simulink library "mbd_s32k_examples"  (Simulink 9.0)
settings: Solver=FixedStepDiscrete  StartTime=0.0  StopTime=10.0  FixedStep=0.1  RelTol=1e-3  EnableMultiTasking=on
InitFcn:
  | mbd_s32k14_consistency_checks(bdroot(gcs));
(part 2 of 3)

== system mbd_s32k_examples/S32K11x MCU Simulink Models/Communications Modules/CAN ==
  CAN_Echo : Subsystem  mask{A=[]}
      mask prompts: A "Needed to invoke OpenFcn from the browser:"
      settings: OpenFcn=sfundemo_open('flexcan_echo_s32k11x')
      mask Display: disp('FlexCAN\nEcho');
  CAN_FD_Master : Subsystem  mask{A=[]}
      mask prompts: A "Needed to invoke OpenFcn from the browser:"
      settings: OpenFcn=sfundemo_open('flexcan_can_fd_master_s32k11x')
      mask Display: disp('FlexCAN\nFD Master');
  CAN_FD_Slave : Subsystem  mask{A=[]}
      mask prompts: A "Needed to invoke OpenFcn from the browser:"
      settings: OpenFcn=sfundemo_open('flexcan_can_fd_slave_s32k11x')
      mask Display: disp('FlexCAN\nFD Slave');
  CAN_Loopback : Subsystem  mask{A=[]}
      mask prompts: A "Needed to invoke OpenFcn from the browser:"
      settings: OpenFcn=sfundemo_open('flexcan_loopback_s32k11x')
      mask Display: disp('FlexCAN\nLoopback');
  CAN_Master_XFER : Subsystem  mask{A=[]}
      mask prompts: A "Needed to invoke OpenFcn from the browser:"
      settings: OpenFcn=sfundemo_open('flexcan_master_xfer_status_s32k11x')
      mask Display: disp('FlexCAN\nMaster XFER');
  CAN_Traffic : Subsystem  mask{A=[]}
      mask prompts: A "Needed to invoke OpenFcn from the browser:"
      settings: OpenFcn=sfundemo_open('flexcan_s32k11x')
      mask Display: disp('FlexCAN\nTraffic');

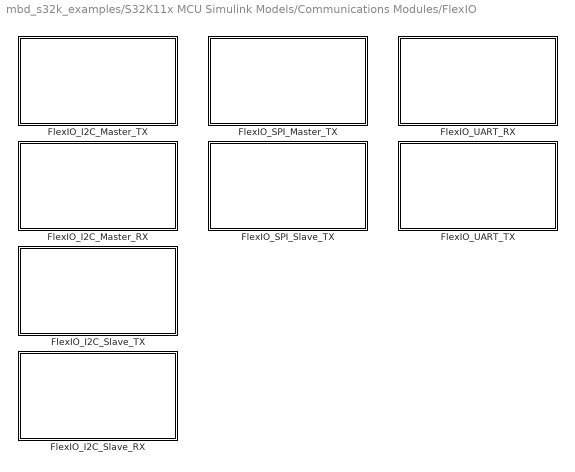
== system mbd_s32k_examples/S32K11x MCU Simulink Models/Communications Modules/FlexIO ==
  FlexIO_I2C_Master_RX : Subsystem  mask{A=[]}
      mask prompts: A "Needed to invoke OpenFcn from the browser:"
      settings: OpenFcn=sfundemo_open('fxio_i2c_master_rx_s32k11x')
      mask Display: disp('FlexIO I2C\nMaster Receive');
  FlexIO_I2C_Master_TX : Subsystem  mask{A=[]}
      mask prompts: A "Needed to invoke OpenFcn from the browser:"
      settings: OpenFcn=sfundemo_open('fxio_i2c_master_tx_s32k11x')
      mask Display: disp('FlexIO I2C\nMaster Transfer');
  FlexIO_I2C_Slave_RX : Subsystem  mask{A=[]}
      mask prompts: A "Needed to invoke OpenFcn from the browser:"
      settings: OpenFcn=sfundemo_open('fxio_i2c_slave_rx_s32k11x')
      mask Display: disp('FlexIO I2C\nSlave Receive');
  FlexIO_I2C_Slave_TX : Subsystem  mask{A=[]}
      mask prompts: A "Needed to invoke OpenFcn from the browser:"
      settings: OpenFcn=sfundemo_open('fxio_i2c_slave_tx_s32k11x')
      mask Display: disp('FlexIO I2C\nSlave Transfer');
  FlexIO_SPI_Master_TX : Subsystem  mask{A=[]}
      mask prompts: A "Needed to invoke OpenFcn from the browser:"
      settings: OpenFcn=sfundemo_open('fxio_spi_master_s32k11x')
      mask Display: disp('FlexIO SPI\nMaster Transfer');
  FlexIO_SPI_Slave_TX : Subsystem  mask{A=[]}
      mask prompts: A "Needed to invoke OpenFcn from the browser:"
      settings: OpenFcn=sfundemo_open('fxio_spi_slave_s32k11x')
      mask Display: disp('FlexIO SPI\nSlave Transfer');
  FlexIO_UART_RX : Subsystem  mask{A=[]}
      mask prompts: A "Needed to invoke OpenFcn from the browser:"
      settings: OpenFcn=sfundemo_open('fxio_uart_receive_isr_s32k11x')
      mask Display: disp('FlexIO UART\nRX');
  FlexIO_UART_TX : Subsystem  mask{A=[]}
      mask prompts: A "Needed to invoke OpenFcn from the browser:"
      settings: OpenFcn=sfundemo_open('fxio_uart_transmit_isr_s32k11x')
      mask Display: disp('FlexIO UART\nTX');

== system mbd_s32k_examples/S32K11x MCU Simulink Models/Communications Modules/I2C ==
  I2C_Master_Request : Subsystem  mask{A=[]}
      mask prompts: A "Needed to invoke OpenFcn from the browser:"
      settings: OpenFcn=sfundemo_open('lpi2c_master_request_s32k11x')
      mask Display: disp('I2C\nMaster Request');
  I2C_Master_Send : Subsystem  mask{A=[]}
      mask prompts: A "Needed to invoke OpenFcn from the browser:"
      settings: OpenFcn=sfundemo_open('lpi2c_master_send_s32k11x')
      mask Display: disp('I2C\nMaster Send');
  I2C_Slave_Receive : Subsystem  mask{A=[]}
      mask prompts: A "Needed to invoke OpenFcn from the browser:"
      settings: OpenFcn=sfundemo_open('lpi2c_slave_recv_s32k11x')
      mask Display: disp('I2C\nSlave Receive');
  I2C_Slave_Send : Subsystem  mask{A=[]}
      mask prompts: A "Needed to invoke OpenFcn from the browser:"
      settings: OpenFcn=sfundemo_open('lpi2c_master_send_s32k11x')
      mask Display: disp('I2C\nSlave Send');

== system mbd_s32k_examples/S32K11x MCU Simulink Models/Communications Modules/SPI ==
  SPI_Master_Slave_Communication : Subsystem  mask{A=[]}
      mask prompts: A "Needed to invoke OpenFcn from the browser:"
      settings: OpenFcn=sfundemo_open('lpspi_master_slave_s32k11x')
      mask Display: disp('SPI\nMaster&Slave\nPing Pong');

== system mbd_s32k_examples/S32K11x MCU Simulink Models/Communications Modules/Serial ==
  UART_Echo : Subsystem  mask{A=[]}
      mask prompts: A "Needed to invoke OpenFcn from the browser:"
      settings: OpenFcn=sfundemo_open('lpuart_s32k11x')
      mask Display: disp('LPUART\nEcho');
  UART_Hello_World : Subsystem  mask{A=[]}
      mask prompts: A "Needed to invoke OpenFcn from the browser:"
      settings: OpenFcn=sfundemo_open('lpuart_hello_world_s32k11x')
      mask Display: disp('UART\nHello World');

== system mbd_s32k_examples/S32K11x MCU Simulink Models/Core & Systems/DMA_Scatter_Gather ==
  Gain : Gain  SaturateOnIntegerOverflow=on  OutDataTypeStr=Inherit: Same as input  ParamDataTypeStr=Inherit: Same as input

== system mbd_s32k_examples/S32K11x MCU Simulink Models/Core & Systems/DMA_Transfer ==
  Gain : Gain  SaturateOnIntegerOverflow=on  OutDataTypeStr=Inherit: Same as input  ParamDataTypeStr=Inherit: Same as input

== system mbd_s32k_examples/S32K11x MCU Simulink Models/Core & Systems/Low_Power_Complex_Counter ==
  Gain : Gain  SaturateOnIntegerOverflow=on  OutDataTypeStr=Inherit: Same as input  ParamDataTypeStr=Inherit: Same as input

== system mbd_s32k_examples/S32K11x MCU Simulink Models/Core & Systems/Low_Power_Pulse_Counter ==
  Gain : Gain  SaturateOnIntegerOverflow=on  OutDataTypeStr=Inherit: Same as input  ParamDataTypeStr=Inherit: Same as input

== system mbd_s32k_examples/S32K11x MCU Simulink Models/Core & Systems/Low_Power_Timer ==
  Gain : Gain  SaturateOnIntegerOverflow=on  OutDataTypeStr=Inherit: Same as input  ParamDataTypeStr=Inherit: Same as input

== system mbd_s32k_examples/S32K11x MCU Simulink Models/Core & Systems/Power_Management_IO ==
  Gain : Gain  SaturateOnIntegerOverflow=on  OutDataTypeStr=Inherit: Same as input  ParamDataTypeStr=Inherit: Same as input

== system mbd_s32k_examples/S32K11x MCU Simulink Models/Core & Systems/Power_Management_ISR ==
  Gain : Gain  SaturateOnIntegerOverflow=on  OutDataTypeStr=Inherit: Same as input  ParamDataTypeStr=Inherit: Same as input

== system mbd_s32k_examples/S32K11x MCU Simulink Models/Core & Systems/Power_Management_Modes ==
  Gain : Gain  SaturateOnIntegerOverflow=on  OutDataTypeStr=Inherit: Same as input  ParamDataTypeStr=Inherit: Same as input

== system mbd_s32k_examples/S32K11x MCU Simulink Models/Core & Systems/RTC_Alarm ==
  Gain : Gain  SaturateOnIntegerOverflow=on  OutDataTypeStr=Inherit: Same as input  ParamDataTypeStr=Inherit: Same as input

== system mbd_s32k_examples/S32K11x MCU Simulink Models/Core & Systems/Watchdog_Reset ==
  Gain : Gain  SaturateOnIntegerOverflow=on  OutDataTypeStr=Inherit: Same as input  ParamDataTypeStr=Inherit: Same as input

== system mbd_s32k_examples/S32K11x MCU Simulink Models/Download in FLASH/FLASH_BAM_S32K116 ==
  Gain : Gain  SaturateOnIntegerOverflow=on  OutDataTypeStr=Inherit: Same as input  ParamDataTypeStr=Inherit: Same as input

== system mbd_s32k_examples/S32K11x MCU Simulink Models/Download in FLASH/FLASH_BAM_S32K118 ==
  Gain : Gain  SaturateOnIntegerOverflow=on  OutDataTypeStr=Inherit: Same as input  ParamDataTypeStr=Inherit: Same as input

== system mbd_s32k_examples/S32K11x MCU Simulink Models/General Purpose IO/GPIO_ISR ==
  Gain : Gain  SaturateOnIntegerOverflow=on  OutDataTypeStr=Inherit: Same as input  ParamDataTypeStr=Inherit: Same as input

== system mbd_s32k_examples/S32K11x MCU Simulink Models/General Purpose IO/GPIO_S32K11xEVB ==
  Gain : Gain  SaturateOnIntegerOverflow=on  OutDataTypeStr=Inherit: Same as input  ParamDataTypeStr=Inherit: Same as input

== system mbd_s32k_examples/S32K11x MCU Simulink Models/Hardware Timers/CAP_Dual_Edge ==
  Gain : Gain  SaturateOnIntegerOverflow=on  OutDataTypeStr=Inherit: Same as input  ParamDataTypeStr=Inherit: Same as input

== system mbd_s32k_examples/S32K11x MCU Simulink Models/Hardware Timers/CAP_Edge ==
  Gain : Gain  SaturateOnIntegerOverflow=on  OutDataTypeStr=Inherit: Same as input  ParamDataTypeStr=Inherit: Same as input

== system mbd_s32k_examples/S32K11x MCU Simulink Models/Hardware Timers/CAP_Quadrature_Counter_Direction ==
  Gain : Gain  SaturateOnIntegerOverflow=on  OutDataTypeStr=Inherit: Same as input  ParamDataTypeStr=Inherit: Same as input

== system mbd_s32k_examples/S32K11x MCU Simulink Models/Hardware Timers/CAP_Quadrature_Phase_Mode ==
  Gain : Gain  SaturateOnIntegerOverflow=on  OutDataTypeStr=Inherit: Same as input  ParamDataTypeStr=Inherit: Same as input

== system mbd_s32k_examples/S32K11x MCU Simulink Models/Hardware Timers/LPIT_Enable_Disable ==
  Gain : Gain  SaturateOnIntegerOverflow=on  OutDataTypeStr=Inherit: Same as input  ParamDataTypeStr=Inherit: Same as input

== system mbd_s32k_examples/S32K11x MCU Simulink Models/Hardware Timers/LPIT_Start_Stop_Modes ==
  Gain : Gain  SaturateOnIntegerOverflow=on  OutDataTypeStr=Inherit: Same as input  ParamDataTypeStr=Inherit: Same as input

== system mbd_s32k_examples/S32K11x MCU Simulink Models/Hardware Timers/LPIT_Timer_Interrupts ==
  Gain : Gain  SaturateOnIntegerOverflow=on  OutDataTypeStr=Inherit: Same as input  ParamDataTypeStr=Inherit: Same as input

== system mbd_s32k_examples/S32K11x MCU Simulink Models/Hardware Timers/PDB_Counter_Interrupts ==
  Gain : Gain  SaturateOnIntegerOverflow=on  OutDataTypeStr=Inherit: Same as input  ParamDataTypeStr=Inherit: Same as input

== system mbd_s32k_examples/S32K11x MCU Simulink Models/Hardware Timers/PWM_Complementary ==
  Gain : Gain  SaturateOnIntegerOverflow=on  OutDataTypeStr=Inherit: Same as input  ParamDataTypeStr=Inherit: Same as input

== system mbd_s32k_examples/S32K11x MCU Simulink Models/Hardware Timers/PWM_Edge_Aligned ==
  Gain : Gain  SaturateOnIntegerOverflow=on  OutDataTypeStr=Inherit: Same as input  ParamDataTypeStr=Inherit: Same as input

== system mbd_s32k_examples/S32K11x MCU Simulink Models/Hardware Timers/PWM_Three_Phase ==
  Gain : Gain  SaturateOnIntegerOverflow=on  OutDataTypeStr=Inherit: Same as input  ParamDataTypeStr=Inherit: Same as input

== system mbd_s32k_examples/S32K11x MCU Simulink Models/Hardware Timers/TOF_Interrupts ==
  Gain : Gain  SaturateOnIntegerOverflow=on  OutDataTypeStr=Inherit: Same as input  ParamDataTypeStr=Inherit: Same as input

== system mbd_s32k_examples/S32K11x MCU Simulink Models/Local Interconnect Network/LIN Master  ==
  Gain : Gain  SaturateOnIntegerOverflow=on  OutDataTypeStr=Inherit: Same as input  ParamDataTypeStr=Inherit: Same as input

== system mbd_s32k_examples/S32K11x MCU Simulink Models/Local Interconnect Network/LIN Slave ==
  Gain : Gain  SaturateOnIntegerOverflow=on  OutDataTypeStr=Inherit: Same as input  ParamDataTypeStr=Inherit: Same as input

== system mbd_s32k_examples/S32K11x MCU Simulink Models/Peripheral Bridge/Memory_Access_RW ==
  Gain : Gain  SaturateOnIntegerOverflow=on  OutDataTypeStr=Inherit: Same as input  ParamDataTypeStr=Inherit: Same as input

== system mbd_s32k_examples/S32K11x MCU Simulink Models/Peripheral Bridge/Register_Access_RW ==
  Gain : Gain  SaturateOnIntegerOverflow=on  OutDataTypeStr=Inherit: Same as input  ParamDataTypeStr=Inherit: Same as input

== system mbd_s32k_examples/S32K11x MCU Simulink Models/System Basis Chips/SBC_RW_Registers ==
  Gain : Gain  SaturateOnIntegerOverflow=on  OutDataTypeStr=Inherit: Same as input  ParamDataTypeStr=Inherit: Same as input

== system mbd_s32k_examples/S32K11x MCU Simulink Models/System Basis Chips/UJA1169_Control ==
  Gain : Gain  SaturateOnIntegerOverflow=on  OutDataTypeStr=Inherit: Same as input  ParamDataTypeStr=Inherit: Same as input

== system mbd_s32k_examples/S32K14x MCU Simulink Models/AMMCLIB/AMCLIB ==
  AMCLIB_BackEMF_OBSERVER_F16 : Subsystem  mask{A=[]}
      mask prompts: A "Needed to invoke OpenFcn from the browser:"
      settings: OpenFcn=sfundemo_open('ammclib_amclib_observer_F16_s32k14x')
      mask Display: disp('OBSERVERS\nBackEMF observer and\nPosition Tracking observer\nexample for F16 datatypes');
  AMCLIB_BackEMF_OBSERVER_F32 : Subsystem  mask{A=[]}
      mask prompts: A "Needed to invoke OpenFcn from the browser:"
      settings: OpenFcn=sfundemo_open('ammclib_amclib_observer_F32_s32k14x')
      mask Display: disp('OBSERVERS\nBackEMF observer and\nPosition Tracking observer\nexample for F32 datatypes');
  AMCLIB_BackEMF_OBSERVER_FLT : Subsystem  mask{A=[]}
      mask prompts: A "Needed to invoke OpenFcn from the browser:"
      settings: OpenFcn=sfundemo_open('ammclib_amclib_observer_FLT_s32k14x')
      mask Display: disp('OBSERVERS\nBackEMF observer and\nPosition Tracking observer\nexample for FLT datatypes');
  AMCLIB_CURRENT_LOOP : Subsystem  mask{A=[]}
      mask prompts: A "Needed to invoke OpenFcn from the browser:"
      settings: OpenFcn=sfundemo_open('ammclib_amclib_current_loop_s32k14x')
      mask Display: disp('CURRENT LOOP\nCurrent Loop FOC\n for F16/F32/FLT datatypes');
  AMCLIB_FW : Subsystem  mask{A=[]}
      mask prompts: A "Needed to invoke OpenFcn from the browser:"
      settings: OpenFcn=sfundemo_open('ammclib_amclib_field_weakening_s32k14x')
      mask Display: disp('FW\nField-Weakening Algorithm\non PMSM examples\n for F16/F32/FLT datatypes');
  AMCLIB_SPEED_LOOP : Subsystem  mask{A=[]}
      mask prompts: A "Needed to invoke OpenFcn from the browser:"
      settings: OpenFcn=sfundemo_open('ammclib_amclib_speed_loop_s32k14x')
      mask Display: disp('SPEED LOOP\nSpeed Loop FOC\n for F16/F32/FLT datatypes');
  AMCLIB_SPEED_LOOP_with_FW : Subsystem  mask{A=[]}
      mask prompts: A "Needed to invoke OpenFcn from the browser:"
      settings: OpenFcn=sfundemo_open('ammclib_amclib_FW_speed_loop_s32k14x')
      mask Display: disp('FW SPEED LOOP\nSpeed Loop with\nField Weakening examples\nfor F16/F32/FLT datatypes');

== system mbd_s32k_examples/S32K14x MCU Simulink Models/AMMCLIB/GDFLIB ==
  GDFLIB_FIR : Subsystem  mask{A=[]}
      mask prompts: A "Needed to invoke OpenFcn from the browser:"
      settings: OpenFcn=sfundemo_open('ammclib_gdflib_fir_s32k14x')
      mask Display: disp('FIR\nFinite Impulse Response filter for\nF16/F32/FLT datatypes');
  GDFLIB_IIR1 : Subsystem  mask{A=[]}
      mask prompts: A "Needed to invoke OpenFcn from the browser:"
      settings: OpenFcn=sfundemo_open('ammclib_gdflib_iir1_s32k14x')
      mask Display: disp('IIR1\nFirst order\nInfinite Impulse Response filter for\nF16/F32/FLT datatypes');
  GDFLIB_IIR2 : Subsystem  mask{A=[]}
      mask prompts: A "Needed to invoke OpenFcn from the browser:"
      settings: OpenFcn=sfundemo_open('ammclib_gdflib_iir2_s32k14x')
      mask Display: disp('IIR2\nSecond order\nInfinite Impulse Response filter for\nF16/F32/FLT datatypes');
  GDFLIB_MA : Subsystem  mask{A=[]}
      mask prompts: A "Needed to invoke OpenFcn from the browser:"
      settings: OpenFcn=sfundemo_open('ammclib_gdflib_ma_s32k14x')
      mask Display: disp('MA\nMoving Average filter for\nF16/F32/FLT datatypes');

== system mbd_s32k_examples/S32K14x MCU Simulink Models/AMMCLIB/GFLIB ==
  GFLIB_LIMIT : Subsystem  mask{A=[]}
      mask prompts: A "Needed to invoke OpenFcn from the browser:"
      settings: OpenFcn=sfundemo_open('ammclib_gflib_limit_s32k14x')
      mask Display: disp('LIMIT\nScalar and Vector\nlimiting examples for\nF16/F32/FLT datatypes');
  GFLIB_LOG : Subsystem  mask{A=[]}
      mask prompts: A "Needed to invoke OpenFcn from the browser:"
      settings: OpenFcn=sfundemo_open('ammclib_gflib_log_s32k14x')
      mask Display: disp('LOG\nLogarithm examples for\nF16/F32/FLT datatypes');
  GFLIB_LUT : Subsystem  mask{A=[]}
      mask prompts: A "Needed to invoke OpenFcn from the browser:"
      settings: OpenFcn=sfundemo_open('ammclib_gflib_lut_s32k14x')
      mask Display: disp('LUT\nLook-up-Tables examples for\nF16/F32/FLT datatypes');
  GFLIB_MISCELLANEOUS : Subsystem  mask{A=[]}
      mask prompts: A "Needed to invoke OpenFcn from the browser:"
      settings: OpenFcn=sfundemo_open('ammclib_gflib_miscellaneous_s32k14x')
      mask Display: disp('MISC\nSQRT/SIGN/INT/RAMP/HYST\n examples for\nF16/F32/FLT datatypes');
  GFLIB_PIP : Subsystem  mask{A=[]}
      mask prompts: A "Needed to invoke OpenFcn from the browser:"
      settings: OpenFcn=sfundemo_open('ammclib_gflib_pip_s32k14x')
      mask Display: disp('PIp\nPI parallel form examples for\nF16/F32/FLT datatypes');
  GFLIB_PIR : Subsystem  mask{A=[]}
      mask prompts: A "Needed to invoke OpenFcn from the browser:"
      settings: OpenFcn=sfundemo_open('ammclib_gflib_pir_s32k14x')
      mask Display: disp('PIr\nPI reccurent form examples for\nF16/F32/FLT datatypes');
  GFLIB_TRIGONOMETRIC : Subsystem  mask{A=[]}
      mask prompts: A "Needed to invoke OpenFcn from the browser:"
      settings: OpenFcn=sfundemo_open('ammclib_gflib_trigonometric_s32k14x')
      mask Display: disp('TRIGONOMETRIC\nTrigonometric SIN/COS/TAN\n examples for\nF16/F32/FLT datatypes');

== system mbd_s32k_examples/S32K14x MCU Simulink Models/AMMCLIB/GMCLIB ==
  GMCLIB_FOC_F16 : Subsystem  mask{A=[]}
      mask prompts: A "Needed to invoke OpenFcn from the browser:"
      settings: OpenFcn=sfundemo_open('ammclib_gmclib_foc_F16_s32k14x')
      mask Display: disp('FOC\nField Oriented Control\nCoordinate Transformations and\nPWM signal generation\nexample for\nF16 datatypes');
  GMCLIB_FOC_F32 : Subsystem  mask{A=[]}
      mask prompts: A "Needed to invoke OpenFcn from the browser:"
      settings: OpenFcn=sfundemo_open('ammclib_gmclib_foc_F32_s32k14x')
      mask Display: disp('FOC\nField Oriented Control\nCoordinate Transformations and\nPWM signal generation\nexample for\nF32 datatypes');
  GMCLIB_FOC_FLT : Subsystem  mask{A=[]}
      mask prompts: A "Needed to invoke OpenFcn from the browser:"
      settings: OpenFcn=sfundemo_open('ammclib_gmclib_foc_FLT_s32k14x')
      mask Display: disp('FOC\nField Oriented Control\nCoordinate Transformations and\nPWM signal generation\nexample for\nFLT datatypes');

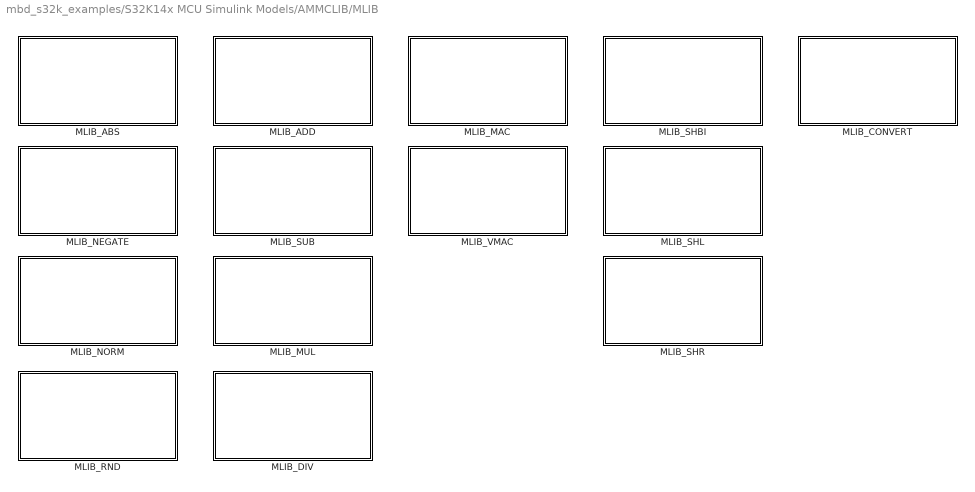
== system mbd_s32k_examples/S32K14x MCU Simulink Models/AMMCLIB/MLIB ==
  MLIB_ABS : Subsystem  mask{A=[]}
      mask prompts: A "Needed to invoke OpenFcn from the browser:"
      settings: OpenFcn=sfundemo_open('ammclib_mlib_abs_s32k14x')
      mask Display: disp('ABS\nModulo examples for\nF16/F32/FLT datatypes');
  MLIB_ADD : Subsystem  mask{A=[]}
      mask prompts: A "Needed to invoke OpenFcn from the browser:"
      settings: OpenFcn=sfundemo_open('ammclib_mlib_add_s32k14x')
      mask Display: disp('ADD\nAddition examples for\nF16/F32/FLT datatypes');
  MLIB_CONVERT : Subsystem  mask{A=[]}
      mask prompts: A "Needed to invoke OpenFcn from the browser:"
      settings: OpenFcn=sfundemo_open('ammclib_mlib_convert_s32k14x')
      mask Display: disp('CONVERT\nType conversions for\nF16/F32/FLT datatypes');
  MLIB_DIV : Subsystem  mask{A=[]}
      mask prompts: A "Needed to invoke OpenFcn from the browser:"
      settings: OpenFcn=sfundemo_open('ammclib_mlib_div_s32k14x')
      mask Display: disp('DIV\nDivision examples for\nF16/F32/FLT datatypes');
  MLIB_MAC : Subsystem  mask{A=[]}
      mask prompts: A "Needed to invoke OpenFcn from the browser:"
      settings: OpenFcn=sfundemo_open('ammclib_mlib_mac_s32k14x')
      mask Display: disp('MAC\nMultiplication with\n Addition/Substraction examples for\nF16/F32/FLT datatypes');
  MLIB_MUL : Subsystem  mask{A=[]}
      mask prompts: A "Needed to invoke OpenFcn from the browser:"
      settings: OpenFcn=sfundemo_open('ammclib_mlib_mul_s32k14x')
      mask Display: disp('MUL\nMultiplication examples for\nF16/F32/FLT datatypes');
  MLIB_NEGATE : Subsystem  mask{A=[]}
      mask prompts: A "Needed to invoke OpenFcn from the browser:"
      settings: OpenFcn=sfundemo_open('ammclib_mlib_neg_s32k14x')
      mask Display: disp('NEGATE\nNegate examples for\nF16/F32/FLT datatypes');
  MLIB_NORM : Subsystem  mask{A=[]}
      mask prompts: A "Needed to invoke OpenFcn from the browser:"
      settings: OpenFcn=sfundemo_open('ammclib_mlib_norm_s32k14x')
      mask Display: disp('NORM\nNormalization examples for\nF16/F32/FLT datatypes');
  MLIB_RND : Subsystem  mask{A=[]}
      mask prompts: A "Needed to invoke OpenFcn from the browser:"
      settings: OpenFcn=sfundemo_open('ammclib_mlib_rnd_s32k14x')
      mask Display: disp('RND\nRound examples for\nF16/F32/FLT datatypes');
  MLIB_SHBI : Subsystem  mask{A=[]}
      mask prompts: A "Needed to invoke OpenFcn from the browser:"
      settings: OpenFcn=sfundemo_open('ammclib_mlib_shbi_s32k14x')
      mask Display: disp('SHBI\nBidirectional Shift examples for\nF16/F32/FLT datatypes');
  MLIB_SHL : Subsystem  mask{A=[]}
      mask prompts: A "Needed to invoke OpenFcn from the browser:"
      settings: OpenFcn=sfundemo_open('ammclib_mlib_shl_s32k14x')
      mask Display: disp('SHL\nLeft Shift examples for\nF16/F32/FLT datatypes');
  MLIB_SHR : Subsystem  mask{A=[]}
      mask prompts: A "Needed to invoke OpenFcn from the browser:"
      settings: OpenFcn=sfundemo_open('ammclib_mlib_shr_s32k14x')
      mask Display: disp('SHR\nRight Shift examples for\nF16/F32/FLT datatypes');
  MLIB_SUB : Subsystem  mask{A=[]}
      mask prompts: A "Needed to invoke OpenFcn from the browser:"
      settings: OpenFcn=sfundemo_open('ammclib_mlib_sub_s32k14x')
      mask Display: disp('SUB\nSubstraction examples for\nF16/F32/FLT datatypes');
  MLIB_VMAC : Subsystem  mask{A=[]}
      mask prompts: A "Needed to invoke OpenFcn from the browser:"
      settings: OpenFcn=sfundemo_open('ammclib_mlib_vmac_s32k14x')
      mask Display: disp('VMAC\nVector multiplication examples for\nF16/F32/FLT datatypes');

== system mbd_s32k_examples/S32K14x MCU Simulink Models/Analog/ADC_Hardware_Triggered ==
  Gain : Gain  SaturateOnIntegerOverflow=on  OutDataTypeStr=Inherit: Same as input  ParamDataTypeStr=Inherit: Same as input

== system mbd_s32k_examples/S32K14x MCU Simulink Models/Analog/ADC_Potentiometer ==
  Gain : Gain  SaturateOnIntegerOverflow=on  OutDataTypeStr=Inherit: Same as input  ParamDataTypeStr=Inherit: Same as input

== system mbd_s32k_examples/S32K14x MCU Simulink Models/Analog/ADC_Software_Triggered ==
  Gain : Gain  SaturateOnIntegerOverflow=on  OutDataTypeStr=Inherit: Same as input  ParamDataTypeStr=Inherit: Same as input

== system mbd_s32k_examples/S32K14x MCU Simulink Models/Analog/CMP_IO_Triggering ==
  Gain : Gain  SaturateOnIntegerOverflow=on  OutDataTypeStr=Inherit: Same as input  ParamDataTypeStr=Inherit: Same as input

== system mbd_s32k_examples/S32K14x MCU Simulink Models/Analog/FTM_PDB_ADC_Sync_Chaining ==
  Gain : Gain  SaturateOnIntegerOverflow=on  OutDataTypeStr=Inherit: Same as input  ParamDataTypeStr=Inherit: Same as input

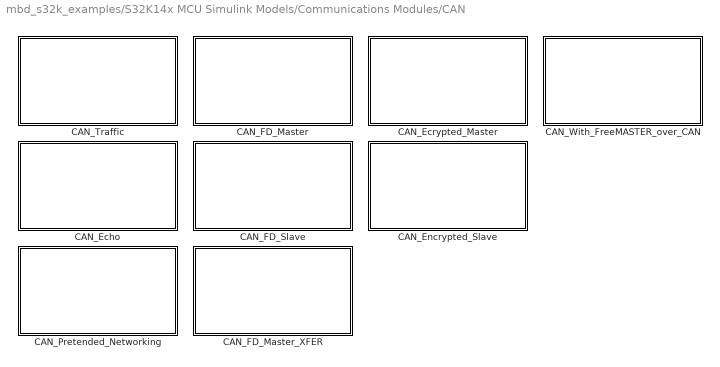
== system mbd_s32k_examples/S32K14x MCU Simulink Models/Communications Modules/CAN ==
  CAN_Echo : Subsystem  mask{A=[]}
      mask prompts: A "Needed to invoke OpenFcn from the browser:"
      settings: OpenFcn=sfundemo_open('flexcan_echo_s32k14x')
      mask Display: disp('FlexCAN\nEcho');
  CAN_Ecrypted_Master : Subsystem  mask{A=[]}
      mask prompts: A "Needed to invoke OpenFcn from the browser:"
      settings: OpenFcn=sfundemo_open('flexcan_encrypted_master_s32k14x')
      mask Display: disp('FlexCAN\nEncrypted Master');
  CAN_Encrypted_Slave : Subsystem  mask{A=[]}
      mask prompts: A "Needed to invoke OpenFcn from the browser:"
      settings: OpenFcn=sfundemo_open('flexcan_encrypted_slave_s32k14x')
      mask Display: disp('FlexCAN\nEncrypted Slave');
  CAN_FD_Master : Subsystem  mask{A=[]}
      mask prompts: A "Needed to invoke OpenFcn from the browser:"
      settings: OpenFcn=sfundemo_open('flexcan_can_fd_master_s32k14x')
      mask Display: disp('FlexCAN\nFD Master');
  CAN_FD_Master_XFER : Subsystem  mask{A=[]}
      mask prompts: A "Needed to invoke OpenFcn from the browser:"
      settings: OpenFcn=sfundemo_open('flexcan_fd_master_xfer_status_s32k14x')
      mask Display: disp('FlexCAN\nFD Master XFER');
  CAN_FD_Slave : Subsystem  mask{A=[]}
      mask prompts: A "Needed to invoke OpenFcn from the browser:"
      settings: OpenFcn=sfundemo_open('flexcan_can_fd_slave_s32k14x')
      mask Display: disp('FlexCAN\nFD Slave');
  CAN_Pretended_Networking : Subsystem  mask{A=[]}
      mask prompts: A "Needed to invoke OpenFcn from the browser:"
      settings: OpenFcn=sfundemo_open('flexcan_pnet_s32k14x')
      mask Display: disp('FlexCAN\nPretended Networking');
  CAN_Traffic : Subsystem  mask{A=[]}
      mask prompts: A "Needed to invoke OpenFcn from the browser:"
      settings: OpenFcn=sfundemo_open('flexcan_s32k14x')
      mask Display: disp('FlexCAN\nTraffic');
  CAN_With_FreeMASTER_over_CAN : Subsystem  mask{A=[]}
      mask prompts: A "Needed to invoke OpenFcn from the browser:"
      settings: OpenFcn=sfundemo_open('flexcan_and_fm_over_can_s32k14x')
      mask Display: disp('FlexCAN\nWith FreeMASTER over CAN');

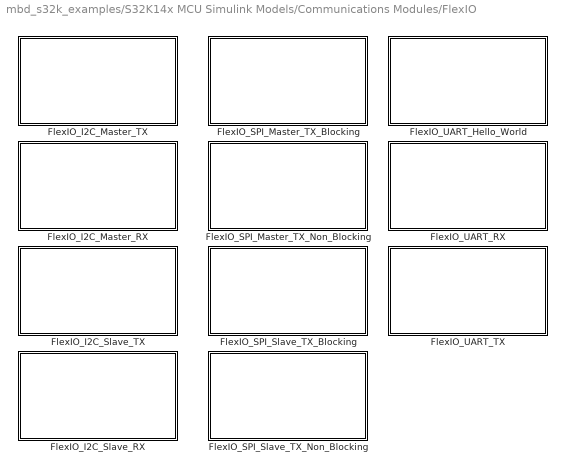
== system mbd_s32k_examples/S32K14x MCU Simulink Models/Communications Modules/FlexIO ==
  FlexIO_I2C_Master_RX : Subsystem  mask{A=[]}
      mask prompts: A "Needed to invoke OpenFcn from the browser:"
      settings: OpenFcn=sfundemo_open('fxio_i2c_master_rx_s32k14x')
      mask Display: disp('FlexIO I2C\nMaster Receive');
  FlexIO_I2C_Master_TX : Subsystem  mask{A=[]}
      mask prompts: A "Needed to invoke OpenFcn from the browser:"
      settings: OpenFcn=sfundemo_open('fxio_i2c_master_tx_s32k14x')
      mask Display: disp('FlexIO I2C\nMaster Transfer');
  FlexIO_I2C_Slave_RX : Subsystem  mask{A=[]}
      mask prompts: A "Needed to invoke OpenFcn from the browser:"
      settings: OpenFcn=sfundemo_open('fxio_i2c_slave_rx_s32k14x')
      mask Display: disp('FlexIO I2C\nSlave Receive');
  FlexIO_I2C_Slave_TX : Subsystem  mask{A=[]}
      mask prompts: A "Needed to invoke OpenFcn from the browser:"
      settings: OpenFcn=sfundemo_open('fxio_i2c_slave_tx_s32k14x')
      mask Display: disp('FlexIO I2C\nSlave Transfer');
  FlexIO_SPI_Master_TX_Blocking : Subsystem  mask{A=[]}
      mask prompts: A "Needed to invoke OpenFcn from the browser:"
      settings: OpenFcn=sfundemo_open('fxio_spi_master_blocking_s32k14x')
      mask Display: disp('FlexIO SPI\nMaster Transfer blocking');
  FlexIO_SPI_Master_TX_Non_Blocking : Subsystem  mask{A=[]}
      mask prompts: A "Needed to invoke OpenFcn from the browser:"
      settings: OpenFcn=sfundemo_open('fxio_spi_master_non_blocking_s32k14x')
      mask Display: disp('FlexIO SPI\nMaster Transfer non blocking');
  FlexIO_SPI_Slave_TX_Blocking : Subsystem  mask{A=[]}
      mask prompts: A "Needed to invoke OpenFcn from the browser:"
      settings: OpenFcn=sfundemo_open('fxio_spi_slave_blocking_s32k14x')
      mask Display: disp('FlexIO SPI\nSlave Transfer blocking');
  FlexIO_SPI_Slave_TX_Non_Blocking : Subsystem  mask{A=[]}
      mask prompts: A "Needed to invoke OpenFcn from the browser:"
      settings: OpenFcn=sfundemo_open('fxio_spi_slave_non_blocking_s32k14x')
      mask Display: disp('FlexIO SPI\nSlave Transfer non blocking');
  FlexIO_UART_Hello_World : Subsystem  mask{A=[]}
      mask prompts: A "Needed to invoke OpenFcn from the browser:"
      settings: OpenFcn=sfundemo_open('fxio_uart_hello_world_s32k14x')
      mask Display: disp('FlexIO UART\nHello World');
  FlexIO_UART_RX : Subsystem  mask{A=[]}
      mask prompts: A "Needed to invoke OpenFcn from the browser:"
      settings: OpenFcn=sfundemo_open('fxio_uart_receive_isr_s32k14x')
      mask Display: disp('FlexIO UART\nRX');
  FlexIO_UART_TX : Subsystem  mask{A=[]}
      mask prompts: A "Needed to invoke OpenFcn from the browser:"
      settings: OpenFcn=sfundemo_open('fxio_uart_transmit_isr_s32k14x')
      mask Display: disp('FlexIO UART\nTX');

== system mbd_s32k_examples/S32K14x MCU Simulink Models/Communications Modules/I2C ==
  I2C_Master_Request : Subsystem  mask{A=[]}
      mask prompts: A "Needed to invoke OpenFcn from the browser:"
      settings: OpenFcn=sfundemo_open('lpi2c_master_request_s32k14x')
      mask Display: disp('I2C\nMaster Request');
  I2C_Master_Send : Subsystem  mask{A=[]}
      mask prompts: A "Needed to invoke OpenFcn from the browser:"
      settings: OpenFcn=sfundemo_open('lpi2c_master_send_s32k14x')
      mask Display: disp('I2C\nMaster Send');
  I2C_Slave_Receive : Subsystem  mask{A=[]}
      mask prompts: A "Needed to invoke OpenFcn from the browser:"
      settings: OpenFcn=sfundemo_open('lpi2c_slave_recv_s32k14x')
      mask Display: disp('I2C\nSlave Receive');
  I2C_Slave_Send : Subsystem  mask{A=[]}
      mask prompts: A "Needed to invoke OpenFcn from the browser:"
      settings: OpenFcn=sfundemo_open('lpi2c_master_send_s32k14x')
      mask Display: disp('I2C\nSlave Send');

== system mbd_s32k_examples/S32K14x MCU Simulink Models/Communications Modules/SPI ==
  SPI_Master_Slave_Communication : Subsystem  mask{A=[]}
      mask prompts: A "Needed to invoke OpenFcn from the browser:"
      settings: OpenFcn=sfundemo_open('lpspi_master_slave_s32k14x')
      mask Display: disp('SPI\nMaster&Slave\nPing Pong');

== system mbd_s32k_examples/S32K14x MCU Simulink Models/Communications Modules/Serial ==
  UART_Echo : Subsystem  mask{A=[]}
      mask prompts: A "Needed to invoke OpenFcn from the browser:"
      settings: OpenFcn=sfundemo_open('lpuart_s32k14x')
      mask Display: disp('LPUART\nEcho');
  UART_Hello_World : Subsystem  mask{A=[]}
      mask prompts: A "Needed to invoke OpenFcn from the browser:"
      settings: OpenFcn=sfundemo_open('lpuart_hello_world_s32k14x')
      mask Display: disp('UART\nHello World');
  UART_Relay : Subsystem  mask{A=[]}
      mask prompts: A "Needed to invoke OpenFcn from the browser:"
      settings: OpenFcn=sfundemo_open('lpuart_relay_s32k14x')
      mask Display: disp('LPUART\nRelay');

== system mbd_s32k_examples/S32K14x MCU Simulink Models/Core & Systems/CSEC_Encrypt_Decrypt ==
  Gain : Gain  SaturateOnIntegerOverflow=on  OutDataTypeStr=Inherit: Same as input  ParamDataTypeStr=Inherit: Same as input

== system mbd_s32k_examples/S32K14x MCU Simulink Models/Core & Systems/DMA_Block_Transfer ==
  Gain : Gain  SaturateOnIntegerOverflow=on  OutDataTypeStr=Inherit: Same as input  ParamDataTypeStr=Inherit: Same as input

== system mbd_s32k_examples/S32K14x MCU Simulink Models/Core & Systems/DMA_Scatter_Gather ==
  Gain : Gain  SaturateOnIntegerOverflow=on  OutDataTypeStr=Inherit: Same as input  ParamDataTypeStr=Inherit: Same as input

== system mbd_s32k_examples/S32K14x MCU Simulink Models/Core & Systems/DMA_Transfer ==
  Gain : Gain  SaturateOnIntegerOverflow=on  OutDataTypeStr=Inherit: Same as input  ParamDataTypeStr=Inherit: Same as input

== system mbd_s32k_examples/S32K14x MCU Simulink Models/Core & Systems/Low_Power_Complex_Counter ==
  Gain : Gain  SaturateOnIntegerOverflow=on  OutDataTypeStr=Inherit: Same as input  ParamDataTypeStr=Inherit: Same as input

== system mbd_s32k_examples/S32K14x MCU Simulink Models/Core & Systems/Low_Power_Pulse_Counter ==
  Gain : Gain  SaturateOnIntegerOverflow=on  OutDataTypeStr=Inherit: Same as input  ParamDataTypeStr=Inherit: Same as input

== system mbd_s32k_examples/S32K14x MCU Simulink Models/Core & Systems/Low_Power_Timer ==
  Gain : Gain  SaturateOnIntegerOverflow=on  OutDataTypeStr=Inherit: Same as input  ParamDataTypeStr=Inherit: Same as input

== system mbd_s32k_examples/S32K14x MCU Simulink Models/Core & Systems/Power_Management_IO ==
  Gain : Gain  SaturateOnIntegerOverflow=on  OutDataTypeStr=Inherit: Same as input  ParamDataTypeStr=Inherit: Same as input

== system mbd_s32k_examples/S32K14x MCU Simulink Models/Core & Systems/Power_Management_ISR ==
  Gain : Gain  SaturateOnIntegerOverflow=on  OutDataTypeStr=Inherit: Same as input  ParamDataTypeStr=Inherit: Same as input

== system mbd_s32k_examples/S32K14x MCU Simulink Models/Core & Systems/Power_Management_Modes ==
  Gain : Gain  SaturateOnIntegerOverflow=on  OutDataTypeStr=Inherit: Same as input  ParamDataTypeStr=Inherit: Same as input

== system mbd_s32k_examples/S32K14x MCU Simulink Models/Core & Systems/Power_Management_Sleep ==
  Gain : Gain  SaturateOnIntegerOverflow=on  OutDataTypeStr=Inherit: Same as input  ParamDataTypeStr=Inherit: Same as input

== system mbd_s32k_examples/S32K14x MCU Simulink Models/Core & Systems/RTC_Alarm ==
  Gain : Gain  SaturateOnIntegerOverflow=on  OutDataTypeStr=Inherit: Same as input  ParamDataTypeStr=Inherit: Same as input

== system mbd_s32k_examples/S32K14x MCU Simulink Models/Core & Systems/Watchdog_Reset ==
  Gain : Gain  SaturateOnIntegerOverflow=on  OutDataTypeStr=Inherit: Same as input  ParamDataTypeStr=Inherit: Same as input

== system mbd_s32k_examples/S32K14x MCU Simulink Models/Download in FLASH/FLASH_BAM_S32K142 ==
  Gain : Gain  SaturateOnIntegerOverflow=on  OutDataTypeStr=Inherit: Same as input  ParamDataTypeStr=Inherit: Same as input

== system mbd_s32k_examples/S32K14x MCU Simulink Models/Download in FLASH/FLASH_BAM_S32K144 ==
  Gain : Gain  SaturateOnIntegerOverflow=on  OutDataTypeStr=Inherit: Same as input  ParamDataTypeStr=Inherit: Same as input

== system mbd_s32k_examples/S32K14x MCU Simulink Models/Download in FLASH/FLASH_BAM_S32K146 ==
  Gain : Gain  SaturateOnIntegerOverflow=on  OutDataTypeStr=Inherit: Same as input  ParamDataTypeStr=Inherit: Same as input

== system mbd_s32k_examples/S32K14x MCU Simulink Models/Download in FLASH/FLASH_BAM_S32K148 ==
  Gain : Gain  SaturateOnIntegerOverflow=on  OutDataTypeStr=Inherit: Same as input  ParamDataTypeStr=Inherit: Same as input

== system mbd_s32k_examples/S32K14x MCU Simulink Models/Download in RAM/RAM_BAM_S32K144 ==
  Gain : Gain  SaturateOnIntegerOverflow=on  OutDataTypeStr=Inherit: Same as input  ParamDataTypeStr=Inherit: Same as input

== system mbd_s32k_examples/S32K14x MCU Simulink Models/Download in RAM/RAM_BAM_S32K146 ==
  Gain : Gain  SaturateOnIntegerOverflow=on  OutDataTypeStr=Inherit: Same as input  ParamDataTypeStr=Inherit: Same as input

== system mbd_s32k_examples/S32K14x MCU Simulink Models/Download in RAM/RAM_BAM_S32K148 ==
  Gain : Gain  SaturateOnIntegerOverflow=on  OutDataTypeStr=Inherit: Same as input  ParamDataTypeStr=Inherit: Same as input

== system mbd_s32k_examples/S32K14x MCU Simulink Models/General Purpose IO/GPIO_ISR ==
  Gain : Gain  SaturateOnIntegerOverflow=on  OutDataTypeStr=Inherit: Same as input  ParamDataTypeStr=Inherit: Same as input

== system mbd_s32k_examples/S32K14x MCU Simulink Models/General Purpose IO/GPIO_S32K142EVB ==
  Gain : Gain  SaturateOnIntegerOverflow=on  OutDataTypeStr=Inherit: Same as input  ParamDataTypeStr=Inherit: Same as input

== system mbd_s32k_examples/S32K14x MCU Simulink Models/General Purpose IO/GPIO_S32K144EVB ==
  Gain : Gain  SaturateOnIntegerOverflow=on  OutDataTypeStr=Inherit: Same as input  ParamDataTypeStr=Inherit: Same as input

== system mbd_s32k_examples/S32K14x MCU Simulink Models/General Purpose IO/GPIO_S32K146EVB ==
  Gain : Gain  SaturateOnIntegerOverflow=on  OutDataTypeStr=Inherit: Same as input  ParamDataTypeStr=Inherit: Same as input

== system mbd_s32k_examples/S32K14x MCU Simulink Models/General Purpose IO/GPIO_S32K148EVB ==
  Gain : Gain  SaturateOnIntegerOverflow=on  OutDataTypeStr=Inherit: Same as input  ParamDataTypeStr=Inherit: Same as input

== system mbd_s32k_examples/S32K14x MCU Simulink Models/Hardware Timers/CAP_Dual_Edge ==
  Gain : Gain  SaturateOnIntegerOverflow=on  OutDataTypeStr=Inherit: Same as input  ParamDataTypeStr=Inherit: Same as input

== system mbd_s32k_examples/S32K14x MCU Simulink Models/Hardware Timers/CAP_Edge ==
  Gain : Gain  SaturateOnIntegerOverflow=on  OutDataTypeStr=Inherit: Same as input  ParamDataTypeStr=Inherit: Same as input

== system mbd_s32k_examples/S32K14x MCU Simulink Models/Hardware Timers/CAP_Quadrature_Counter_Direction ==
  Gain : Gain  SaturateOnIntegerOverflow=on  OutDataTypeStr=Inherit: Same as input  ParamDataTypeStr=Inherit: Same as input

== system mbd_s32k_examples/S32K14x MCU Simulink Models/Hardware Timers/CAP_Quadrature_Phase_Mode ==
  Gain : Gain  SaturateOnIntegerOverflow=on  OutDataTypeStr=Inherit: Same as input  ParamDataTypeStr=Inherit: Same as input

== system mbd_s32k_examples/S32K14x MCU Simulink Models/Hardware Timers/LPIT_Enable_Disable ==
  Gain : Gain  SaturateOnIntegerOverflow=on  OutDataTypeStr=Inherit: Same as input  ParamDataTypeStr=Inherit: Same as input

== system mbd_s32k_examples/S32K14x MCU Simulink Models/Hardware Timers/LPIT_Start_Stop_Modes ==
  Gain : Gain  SaturateOnIntegerOverflow=on  OutDataTypeStr=Inherit: Same as input  ParamDataTypeStr=Inherit: Same as input

== system mbd_s32k_examples/S32K14x MCU Simulink Models/Hardware Timers/LPIT_Timer_Interrupts ==
  Gain : Gain  SaturateOnIntegerOverflow=on  OutDataTypeStr=Inherit: Same as input  ParamDataTypeStr=Inherit: Same as input

== system mbd_s32k_examples/S32K14x MCU Simulink Models/Hardware Timers/PDB_Counter_Interrupts ==
  Gain : Gain  SaturateOnIntegerOverflow=on  OutDataTypeStr=Inherit: Same as input  ParamDataTypeStr=Inherit: Same as input

== system mbd_s32k_examples/S32K14x MCU Simulink Models/Hardware Timers/PWM_Complementary ==
  Gain : Gain  SaturateOnIntegerOverflow=on  OutDataTypeStr=Inherit: Same as input  ParamDataTypeStr=Inherit: Same as input

== system mbd_s32k_examples/S32K14x MCU Simulink Models/Hardware Timers/PWM_Edge_Aligned ==
  Gain : Gain  SaturateOnIntegerOverflow=on  OutDataTypeStr=Inherit: Same as input  ParamDataTypeStr=Inherit: Same as input

== system mbd_s32k_examples/S32K14x MCU Simulink Models/Hardware Timers/PWM_Hall_Sensor ==
  Gain : Gain  SaturateOnIntegerOverflow=on  OutDataTypeStr=Inherit: Same as input  ParamDataTypeStr=Inherit: Same as input

== system mbd_s32k_examples/S32K14x MCU Simulink Models/Hardware Timers/PWM_Hall_Sensor_TOF ==
  Gain : Gain  SaturateOnIntegerOverflow=on  OutDataTypeStr=Inherit: Same as input  ParamDataTypeStr=Inherit: Same as input

== system mbd_s32k_examples/S32K14x MCU Simulink Models/Hardware Timers/PWM_Three_Phase ==
  Gain : Gain  SaturateOnIntegerOverflow=on  OutDataTypeStr=Inherit: Same as input  ParamDataTypeStr=Inherit: Same as input

== system mbd_s32k_examples/S32K14x MCU Simulink Models/Hardware Timers/TOF_Interrupts ==
  Gain : Gain  SaturateOnIntegerOverflow=on  OutDataTypeStr=Inherit: Same as input  ParamDataTypeStr=Inherit: Same as input

== system mbd_s32k_examples/S32K14x MCU Simulink Models/Local Interconnect Network/LIN Master  ==
  Gain : Gain  SaturateOnIntegerOverflow=on  OutDataTypeStr=Inherit: Same as input  ParamDataTypeStr=Inherit: Same as input

== system mbd_s32k_examples/S32K14x MCU Simulink Models/Local Interconnect Network/LIN Slave ==
  Gain : Gain  SaturateOnIntegerOverflow=on  OutDataTypeStr=Inherit: Same as input  ParamDataTypeStr=Inherit: Same as input

== system mbd_s32k_examples/S32K14x MCU Simulink Models/Motor Control/6-step commutation sequence based on Hall Sensors transitions  and PI Speed Controller ==
  Gain : Gain  SaturateOnIntegerOverflow=on  OutDataTypeStr=Inherit: Same as input  ParamDataTypeStr=Inherit: Same as input

== system mbd_s32k_examples/S32K14x MCU Simulink Models/Motor Control/6-step commutation sequence  based on Hall Sensors transitions  ==
  Gain : Gain  SaturateOnIntegerOverflow=on  OutDataTypeStr=Inherit: Same as input  ParamDataTypeStr=Inherit: Same as input

== system mbd_s32k_examples/S32K14x MCU Simulink Models/Motor Control/Closed Loop Speed Control with FOC and Speed Estimator Based on Hall Sensors ==
  Gain : Gain  SaturateOnIntegerOverflow=on  OutDataTypeStr=Inherit: Same as input  ParamDataTypeStr=Inherit: Same as input

== system mbd_s32k_examples/S32K14x MCU Simulink Models/Motor Control/FOC Open Loop based on V/f control method ==
  Gain : Gain  SaturateOnIntegerOverflow=on  OutDataTypeStr=Inherit: Same as input  ParamDataTypeStr=Inherit: Same as input

== system mbd_s32k_examples/S32K14x MCU Simulink Models/Motor and Solenoid Drivers/MC34GD3000_Configuration ==
  Gain : Gain  SaturateOnIntegerOverflow=on  OutDataTypeStr=Inherit: Same as input  ParamDataTypeStr=Inherit: Same as input

== system mbd_s32k_examples/S32K14x MCU Simulink Models/Motor and Solenoid Drivers/MC34GD3000_Functional_Mode ==
  Gain : Gain  SaturateOnIntegerOverflow=on  OutDataTypeStr=Inherit: Same as input  ParamDataTypeStr=Inherit: Same as input

== system mbd_s32k_examples/S32K14x MCU Simulink Models/Peripheral Bridge/Memory_Access_RW ==
  Gain : Gain  SaturateOnIntegerOverflow=on  OutDataTypeStr=Inherit: Same as input  ParamDataTypeStr=Inherit: Same as input

== system mbd_s32k_examples/S32K14x MCU Simulink Models/Peripheral Bridge/Register_Access_RW ==
  Gain : Gain  SaturateOnIntegerOverflow=on  OutDataTypeStr=Inherit: Same as input  ParamDataTypeStr=Inherit: Same as input

== system mbd_s32k_examples/S32K14x MCU Simulink Models/System Basis Chips/SBC_RW_Registers ==
  Gain : Gain  SaturateOnIntegerOverflow=on  OutDataTypeStr=Inherit: Same as input  ParamDataTypeStr=Inherit: Same as input

== system mbd_s32k_examples/S32K14x MCU Simulink Models/System Basis Chips/SBC_RW_Registers  ==
  Gain : Gain  SaturateOnIntegerOverflow=on  OutDataTypeStr=Inherit: Same as input  ParamDataTypeStr=Inherit: Same as input

== system mbd_s32k_examples/S32K14x MCU Simulink Models/System Basis Chips/SBC_Write_Registers ==
  Gain : Gain  SaturateOnIntegerOverflow=on  OutDataTypeStr=Inherit: Same as input  ParamDataTypeStr=Inherit: Same as input

== system mbd_s32k_examples/S32K14x MCU Simulink Models/System Basis Chips/UJA113x_Control ==
  Gain : Gain  SaturateOnIntegerOverflow=on  OutDataTypeStr=Inherit: Same as input  ParamDataTypeStr=Inherit: Same as input

== system mbd_s32k_examples/S32K14x MCU Simulink Models/System Basis Chips/UJA1169_Control ==
  Gain : Gain  SaturateOnIntegerOverflow=on  OutDataTypeStr=Inherit: Same as input  ParamDataTypeStr=Inherit: Same as input

== system mbd_s32k_examples/S32K11x MCU Simulink Models/AMMCLIB/AMCLIB/AMCLIB_BackEMF_OBSERVER_F16 ==
  Gain : Gain  SaturateOnIntegerOverflow=on  OutDataTypeStr=Inherit: Same as input  ParamDataTypeStr=Inherit: Same as input

== system mbd_s32k_examples/S32K11x MCU Simulink Models/AMMCLIB/AMCLIB/AMCLIB_BackEMF_OBSERVER_F32 ==
  Gain : Gain  SaturateOnIntegerOverflow=on  OutDataTypeStr=Inherit: Same as input  ParamDataTypeStr=Inherit: Same as input

== system mbd_s32k_examples/S32K11x MCU Simulink Models/AMMCLIB/AMCLIB/AMCLIB_CURRENT_LOOP ==
  Gain : Gain  SaturateOnIntegerOverflow=on  OutDataTypeStr=Inherit: Same as input  ParamDataTypeStr=Inherit: Same as input

== system mbd_s32k_examples/S32K11x MCU Simulink Models/AMMCLIB/AMCLIB/AMCLIB_FW ==
  Gain : Gain  SaturateOnIntegerOverflow=on  OutDataTypeStr=Inherit: Same as input  ParamDataTypeStr=Inherit: Same as input

== system mbd_s32k_examples/S32K11x MCU Simulink Models/AMMCLIB/AMCLIB/AMCLIB_SPEED_LOOP ==
  Gain : Gain  SaturateOnIntegerOverflow=on  OutDataTypeStr=Inherit: Same as input  ParamDataTypeStr=Inherit: Same as input

== system mbd_s32k_examples/S32K11x MCU Simulink Models/AMMCLIB/AMCLIB/AMCLIB_SPEED_LOOP_with_FW ==
  Gain : Gain  SaturateOnIntegerOverflow=on  OutDataTypeStr=Inherit: Same as input  ParamDataTypeStr=Inherit: Same as input

== system mbd_s32k_examples/S32K11x MCU Simulink Models/AMMCLIB/GDFLIB/GDFLIB_FIR ==
  Gain : Gain  SaturateOnIntegerOverflow=on  OutDataTypeStr=Inherit: Same as input  ParamDataTypeStr=Inherit: Same as input

== system mbd_s32k_examples/S32K11x MCU Simulink Models/AMMCLIB/GDFLIB/GDFLIB_IIR1 ==
  Gain : Gain  SaturateOnIntegerOverflow=on  OutDataTypeStr=Inherit: Same as input  ParamDataTypeStr=Inherit: Same as input

== system mbd_s32k_examples/S32K11x MCU Simulink Models/AMMCLIB/GDFLIB/GDFLIB_IIR2 ==
  Gain : Gain  SaturateOnIntegerOverflow=on  OutDataTypeStr=Inherit: Same as input  ParamDataTypeStr=Inherit: Same as input

== system mbd_s32k_examples/S32K11x MCU Simulink Models/AMMCLIB/GDFLIB/GDFLIB_MA ==
  Gain : Gain  SaturateOnIntegerOverflow=on  OutDataTypeStr=Inherit: Same as input  ParamDataTypeStr=Inherit: Same as input

== system mbd_s32k_examples/S32K11x MCU Simulink Models/AMMCLIB/GFLIB/GFLIB_LIMIT ==
  Gain : Gain  SaturateOnIntegerOverflow=on  OutDataTypeStr=Inherit: Same as input  ParamDataTypeStr=Inherit: Same as input

== system mbd_s32k_examples/S32K11x MCU Simulink Models/AMMCLIB/GFLIB/GFLIB_LUT ==
  Gain : Gain  SaturateOnIntegerOverflow=on  OutDataTypeStr=Inherit: Same as input  ParamDataTypeStr=Inherit: Same as input

== system mbd_s32k_examples/S32K11x MCU Simulink Models/AMMCLIB/GFLIB/GFLIB_MISCELLANEOUS ==
  Gain : Gain  SaturateOnIntegerOverflow=on  OutDataTypeStr=Inherit: Same as input  ParamDataTypeStr=Inherit: Same as input

== system mbd_s32k_examples/S32K11x MCU Simulink Models/AMMCLIB/GFLIB/GFLIB_PIP ==
  Gain : Gain  SaturateOnIntegerOverflow=on  OutDataTypeStr=Inherit: Same as input  ParamDataTypeStr=Inherit: Same as input

== system mbd_s32k_examples/S32K11x MCU Simulink Models/AMMCLIB/GFLIB/GFLIB_PIR ==
  Gain : Gain  SaturateOnIntegerOverflow=on  OutDataTypeStr=Inherit: Same as input  ParamDataTypeStr=Inherit: Same as input

== system mbd_s32k_examples/S32K11x MCU Simulink Models/AMMCLIB/GFLIB/GFLIB_TRIGONOMETRIC ==
  Gain : Gain  SaturateOnIntegerOverflow=on  OutDataTypeStr=Inherit: Same as input  ParamDataTypeStr=Inherit: Same as input

== system mbd_s32k_examples/S32K11x MCU Simulink Models/AMMCLIB/GMCLIB/GMCLIB_FOC_F16 ==
  Gain : Gain  SaturateOnIntegerOverflow=on  OutDataTypeStr=Inherit: Same as input  ParamDataTypeStr=Inherit: Same as input

== system mbd_s32k_examples/S32K11x MCU Simulink Models/AMMCLIB/GMCLIB/GMCLIB_FOC_F32 ==
  Gain : Gain  SaturateOnIntegerOverflow=on  OutDataTypeStr=Inherit: Same as input  ParamDataTypeStr=Inherit: Same as input

== system mbd_s32k_examples/S32K11x MCU Simulink Models/AMMCLIB/MLIB/MLIB_ABS ==
  Gain : Gain  SaturateOnIntegerOverflow=on  OutDataTypeStr=Inherit: Same as input  ParamDataTypeStr=Inherit: Same as input

== system mbd_s32k_examples/S32K11x MCU Simulink Models/AMMCLIB/MLIB/MLIB_ADD ==
  Gain : Gain  SaturateOnIntegerOverflow=on  OutDataTypeStr=Inherit: Same as input  ParamDataTypeStr=Inherit: Same as input

== system mbd_s32k_examples/S32K11x MCU Simulink Models/AMMCLIB/MLIB/MLIB_CONVERT ==
  Gain : Gain  SaturateOnIntegerOverflow=on  OutDataTypeStr=Inherit: Same as input  ParamDataTypeStr=Inherit: Same as input

== system mbd_s32k_examples/S32K11x MCU Simulink Models/AMMCLIB/MLIB/MLIB_DIV ==
  Gain : Gain  SaturateOnIntegerOverflow=on  OutDataTypeStr=Inherit: Same as input  ParamDataTypeStr=Inherit: Same as input

== system mbd_s32k_examples/S32K11x MCU Simulink Models/AMMCLIB/MLIB/MLIB_MAC ==
  Gain : Gain  SaturateOnIntegerOverflow=on  OutDataTypeStr=Inherit: Same as input  ParamDataTypeStr=Inherit: Same as input

== system mbd_s32k_examples/S32K11x MCU Simulink Models/AMMCLIB/MLIB/MLIB_MUL ==
  Gain : Gain  SaturateOnIntegerOverflow=on  OutDataTypeStr=Inherit: Same as input  ParamDataTypeStr=Inherit: Same as input

== system mbd_s32k_examples/S32K11x MCU Simulink Models/AMMCLIB/MLIB/MLIB_NEGATE ==
  Gain : Gain  SaturateOnIntegerOverflow=on  OutDataTypeStr=Inherit: Same as input  ParamDataTypeStr=Inherit: Same as input

== system mbd_s32k_examples/S32K11x MCU Simulink Models/AMMCLIB/MLIB/MLIB_NORM ==
  Gain : Gain  SaturateOnIntegerOverflow=on  OutDataTypeStr=Inherit: Same as input  ParamDataTypeStr=Inherit: Same as input

== system mbd_s32k_examples/S32K11x MCU Simulink Models/AMMCLIB/MLIB/MLIB_RND ==
  Gain : Gain  SaturateOnIntegerOverflow=on  OutDataTypeStr=Inherit: Same as input  ParamDataTypeStr=Inherit: Same as input

== system mbd_s32k_examples/S32K11x MCU Simulink Models/AMMCLIB/MLIB/MLIB_SHBI ==
  Gain : Gain  SaturateOnIntegerOverflow=on  OutDataTypeStr=Inherit: Same as input  ParamDataTypeStr=Inherit: Same as input

== system mbd_s32k_examples/S32K11x MCU Simulink Models/AMMCLIB/MLIB/MLIB_SHL ==
  Gain : Gain  SaturateOnIntegerOverflow=on  OutDataTypeStr=Inherit: Same as input  ParamDataTypeStr=Inherit: Same as input

== system mbd_s32k_examples/S32K11x MCU Simulink Models/AMMCLIB/MLIB/MLIB_SHR ==
  Gain : Gain  SaturateOnIntegerOverflow=on  OutDataTypeStr=Inherit: Same as input  ParamDataTypeStr=Inherit: Same as input

== system mbd_s32k_examples/S32K11x MCU Simulink Models/AMMCLIB/MLIB/MLIB_SUB ==
  Gain : Gain  SaturateOnIntegerOverflow=on  OutDataTypeStr=Inherit: Same as input  ParamDataTypeStr=Inherit: Same as input

== system mbd_s32k_examples/S32K11x MCU Simulink Models/AMMCLIB/MLIB/MLIB_VMAC ==
  Gain : Gain  SaturateOnIntegerOverflow=on  OutDataTypeStr=Inherit: Same as input  ParamDataTypeStr=Inherit: Same as input

== system mbd_s32k_examples/S32K11x MCU Simulink Models/Communications Modules/CAN/CAN_Echo ==
  Gain : Gain  SaturateOnIntegerOverflow=on  OutDataTypeStr=Inherit: Same as input  ParamDataTypeStr=Inherit: Same as input

== system mbd_s32k_examples/S32K11x MCU Simulink Models/Communications Modules/CAN/CAN_FD_Master ==
  Gain : Gain  SaturateOnIntegerOverflow=on  OutDataTypeStr=Inherit: Same as input  ParamDataTypeStr=Inherit: Same as input

== system mbd_s32k_examples/S32K11x MCU Simulink Models/Communications Modules/CAN/CAN_FD_Slave ==
  Gain : Gain  SaturateOnIntegerOverflow=on  OutDataTypeStr=Inherit: Same as input  ParamDataTypeStr=Inherit: Same as input
